simulink model "lowpass01"  (R2015a)
settings: Solver=ode45  StartTime=0.0  StopTime=10.0  RelTol=1e-3
undefined symbols (not defined in the file or in its folder): fdesignblkfcn, gcbh
settings Model: Creator=liuqi  LastModifiedBy=liuqi

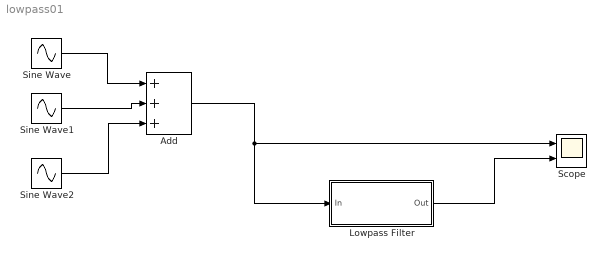
== system lowpass01 ==
  Add : Sum  Inputs=+++
  Lowpass Filter : Subsystem  DialogController=fdesignblkfcn  InitFcn=fdesignblkfcn(gcbh, {'InitFcn'});  mask(Lowpass Filter){}
      mask help: Design a lowpass filter
      settings: CopyFcn=fdesignblkfcn(gcbh, {'CopyFcn'});
      mask Help: helpview(mapfilelocation('dsp'), 'dsplowpassfilter');
      mask Display: disp('Lowpass')
  Scope : Scope  NumInputPorts=2
      settings: YMin=-5~-5  YMax=5~5
  Sine Wave : Sin  Amplitude=10  Frequency=7  SampleTime=0
  Sine Wave1 : Sin  Amplitude=5  Frequency=20  SampleTime=0
  Sine Wave2 : Sin  Amplitude=2  Frequency=35  SampleTime=0
  wires:
  Add/1 -> Scope/1, Lowpass Filter/1(In)
  Lowpass Filter/1(Out) -> Scope/2
  Sine Wave/1 -> Add/1
  Sine Wave1/1 -> Add/2
  Sine Wave2/1 -> Add/3

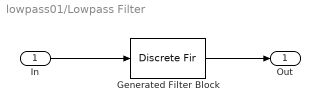
== system lowpass01/Lowpass Filter ==
  In : Inport
  Generated Filter Block : DiscreteFir  Tag=BlockMethodSubSystem  Coefficients=[-0.0034436495845580916 -0.005916479157193442 0.0074434606687912705 0.054740018373940484 0.13478679515848707 0.21479383660135928 0.24873045448052375 0.21479383660135928 0.13478679515848707 0.054740018373940484 0.0074434606687912705 -0.005916479157193442 -0.0034436495845580916]  InputProcessing=Columns as channels (frame based)  SampleTime=0.001
  Out : Outport
  wires:
  In/1 -> Generated Filter Block/1
  Generated Filter Block/1 -> Out/1
